simulink library "pressure_drop_quadratic_fitted_data_water"  (R2018b)
settings: Solver=ode45  StartTime=0.0  StopTime=10.0  RelTol=1e-3  EnableMultiTasking=on
undefined symbols (not defined in the file): acol
settings Model: Creator=lena.frank  LastModifiedBy=drhf
settings DataIOCC: LimitDataPoints=on  SaveFormat=Array  SignalLoggingSaveFormat=ModelDataLogs
settings OptimizationCC: ExpressionDepthLimit=2147483647  LifeSpan=inf
settings DebuggingCC: UnderspecifiedInitializationDetection=Classic  MergeDetectMultiDrivingBlocksExec=none  SolverPrmCheckMsg=warning  FcnCallInpInsideContextMsg=warning  StateNameClashWarn=warning  SFUnexpectedBacktrackingDiag=warning  SFNoUnconditionalDefaultTransitionDiag=warning  SFExecutionAtInitializationDiag=none
settings HardwareCC: ProdBitPerPointer=32  ProdBitPerSizeT=32  ProdBitPerPtrDiffT=32  ProdLargestAtomicFloat=None  ProdIntDivRoundTo=Undefined  ProdEndianess=Unspecified  ProdWordSize=32  ProdHWDeviceType=32-bit Generic
settings ModelReferenceCC: PropagateSignalLabelsOutOfModel=off
settings SFSimCC: SimUseLocalCustomCode=off
settings RTWCC: RTWUseLocalCustomCode=off
settings CodeAppCC: StateflowObjectComments=on
settings GRTTargetCC: TargetLangStandard=C89/C90 (ANSI)  GeneratePreprocessorConditionals=Disable all  CombineOutputUpdateFcns=off  GRTInterface=on
settings ConfigComp: CovMetricSettings=dw  CovHtmlReporting=on  CovSaveCumulativeToWorkspaceVar=on  CovSaveSingleToWorkspaceVar=on  CovExternalEMLEnable=off

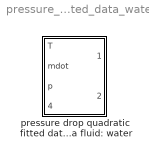
== system pressure_drop_quadratic_fitted_data_water ==
  pressure drop quadratic fitted data fluid: water : Subsystem  mask(pressure drop quadratic fitted data, fluid water){b=0.006201*3.6e4, a=0.000096*1.296e9, aonecol=1.96, acol=acol}
      mask prompts: b "linear term of pressure drop in [Pa/(kg/s)]"; a "quadratic term of pressure drop in [Pa/(kg/s)²]"; aonecol "surface of one collector element in [m²]"; acol "total surface of array (DO NOT CHANGE HERE)"
      mask help:
      | This block calculates the pressure drop of a collector from a fitted parabolic curve. Other temperatures than at test condition (20°C) are interpolated according to a typical pressure drop correlation of a collector for the fluid water.
      | Give parameters in SI-units.
      | Multiply with 3.6e5 to convert from [mbar/(l/h)] to [Pa/(kg/s)].
      | Multiply with 1.296e9 to convert from [mbar/(l/h)²] to [Pa/(kg/s)²].
      | Set "surface of one collector" to the surface of one collector for a parallel arrangement of collectors. Set it to the surface of the array "acol" to model a series arrangement.
      mask Help: web(fullfile(path_carnot('help'),'pressure_drop_quadratic_fitted_data_water.html'),'-helpbrowser')

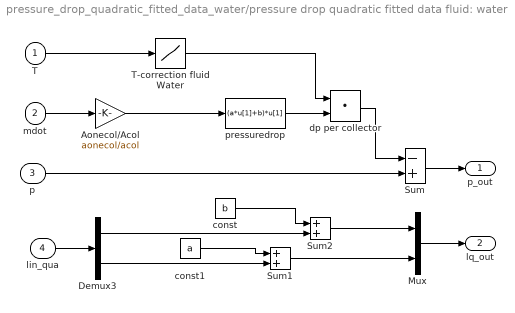
== system pressure_drop_quadratic_fitted_data_water/pressure drop quadratic fitted data fluid: water ==
  T : Inport
  mdot : Inport  Port=2
  p : Inport  Port=3
  lin_qua : Inport  Port=4
  Aonecol/Acol : Gain  Gain=aonecol/acol  SaturateOnIntegerOverflow=on  OutDataTypeStr=Inherit: Same as input  ParamDataTypeStr=Inherit: Same as input
  Demux3 : Demux  Outputs=2
  Mux : Mux  Inputs=2
  Sum : Sum  Inputs=-+  SaturateOnIntegerOverflow=on  InputSameDT=on  OutDataTypeStr=Inherit: Same as first input
  Sum1 : Sum  SaturateOnIntegerOverflow=on  InputSameDT=on  OutDataTypeStr=Inherit: Same as first input
  Sum2 : Sum  SaturateOnIntegerOverflow=on  InputSameDT=on  OutDataTypeStr=Inherit: Same as first input
  T-correction fluid Water : Lookup  InputValues=0:20:200  Table="[0.9985  1.0  1.006  1.0154  1.0275  1.0419  1.0590  1.0794  1.1045  1.1367  1.1795]"  SaturateOnIntegerOverflow=on
  const : Constant  Value=b
  const1 : Constant  Value=a
  dp per collector : DotProduct  InputSameDT=on  OutDataTypeStr=Inherit: Inherit via internal rule
  pressuredrop : Fcn  Expr=(a*u[1]+b)*u[1]
  p_out : Outport
  lq_out : Outport  Port=2
  wires:
  mdot/1 -> Aonecol/Acol/1
  Aonecol/Acol/1 -> pressuredrop/1
  T/1 -> T-correction fluid Water/1
  Sum2/1 -> Mux/1
  const1/1 -> Sum1/1
  const/1 -> Sum2/1
  Demux3/1 -> Sum2/2
  Sum1/1 -> Mux/2
  Sum/1 -> p_out/1
  dp per collector/1 -> Sum/1
  p/1 -> Sum/2
  Mux/1 -> lq_out/1
  Demux3/2 -> Sum1/2
  lin_qua/1 -> Demux3/1
  T-correction fluid Water/1 -> dp per collector/1
  pressuredrop/1 -> dp per collector/2
